simulink model "DSBSC_Modulation"  (R2021a)
settings: Solver=VariableStepAuto  StartTime=0.0  StopTime=10.0  RelTol=1e-3
libraries: dspfdesign x2
settings Model: Creator=ZephyrY  LastModifiedBy=ZephyrY

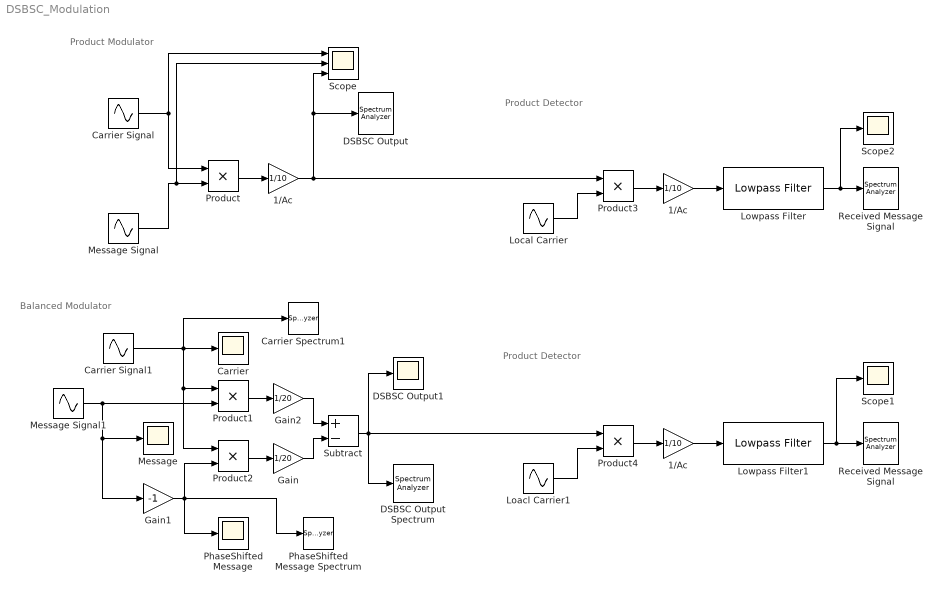
== system DSBSC_Modulation ==
  note: Product Detector
  note: Product Detector
  note: Product Modulator
  note: Balanced Modulator
  1/Ac : Gain  Gain=1/10
  "1/Ac " : Gain  Gain=1/10
  "1/Ac  " : Gain  Gain=1/10
  Carrier : Scope
  Carrier Signal : Sin  Amplitude=10  Frequency=2*pi*100  Phase=pi/2  SampleTime=1e-3
  Carrier Signal1 : Sin  Amplitude=10  Frequency=2*pi*100  Phase=pi/2  SampleTime=1e-3
  Carrier Spectrum1 : SpectrumAnalyzer
  DSBSC Output : SpectrumAnalyzer
  DSBSC Output Spectrum : SpectrumAnalyzer
  DSBSC Output1 : Scope
  Gain : Gain  Gain=1/20
  Gain1 : Gain  Gain=-1
  Gain2 : Gain  Gain=1/20
  Loacl Carrier1 : Sin  Amplitude=10  Frequency=2*pi*100  Phase=pi/2  SampleTime=1e-3
  Local Carrier : Sin  Amplitude=10  Frequency=2*pi*100  Phase=pi/2  SampleTime=1e-3
  Lowpass Filter : dspfdesign/Lowpass Filter  FilterType=FIR  DesignForMinimumOrder=off  FilterOrder=50  PassbandFrequency=15  StopbandFrequency=12e3  PassbandRipple=0.1  StopbandAttenuation=80  InheritSampleRate=on  SampleRate=44100  SimulateUsing=Interpreted execution  roundingMode=Floor  coeffsDataTypeStr=fixdt(1,16)
  Lowpass Filter1 : dspfdesign/Lowpass Filter  FilterType=FIR  DesignForMinimumOrder=off  FilterOrder=50  PassbandFrequency=15  StopbandFrequency=12e3  PassbandRipple=0.1  StopbandAttenuation=80  InheritSampleRate=on  SampleRate=44100  SimulateUsing=Interpreted execution  roundingMode=Floor  coeffsDataTypeStr=fixdt(1,16)
  Message : Scope
  Message Signal : Sin  Amplitude=5  Frequency=2*pi*10  Phase=pi/2  SampleTime=1e-3
  Message Signal1 : Sin  Amplitude=5  Frequency=2*pi*10  Phase=pi/2  SampleTime=1e-3
  PhaseShifted Message : Scope
  PhaseShifted Message Spectrum : SpectrumAnalyzer
  Product{,1..4} (5 alike) : Product
  Received Message Signal : SpectrumAnalyzer
  "Received Message Signal " : SpectrumAnalyzer
  Scope : Scope  NumInputPorts=3
  Scope1 : Scope
  Scope2 : Scope
  Subtract : Sum  Inputs=+-
  wires:
  Carrier Signal/1 -> Scope/1, Product/1
  Message Signal/1 -> Scope/2, Product/2
  Product/1 -> 1/Ac/1
  1/Ac/1 -> DSBSC Output/1, Scope/3, Product3/1
  Gain/1 -> Subtract/2
  Carrier Signal1/1 -> Carrier Spectrum1/1, Product1/1, Product2/1, Carrier/1
  Gain2/1 -> Subtract/1
  Subtract/1 -> DSBSC Output Spectrum/1, Product4/1, DSBSC Output1/1
  Gain1/1 -> PhaseShifted Message Spectrum/1, PhaseShifted Message/1, Product2/2
  Message Signal1/1 -> Product1/2, Gain1/1, Message/1
  Product1/1 -> Gain2/1
  Product2/1 -> Gain/1
  Local Carrier/1 -> Product3/2
  Loacl Carrier1/1 -> Product4/2
  Product3/1 -> "1/Ac  "/1
  Product4/1 -> "1/Ac "/1
  "1/Ac  "/1 -> Lowpass Filter/1
  "1/Ac "/1 -> Lowpass Filter1/1
  Lowpass Filter/1 -> Scope2/1, Received Message Signal/1
  Lowpass Filter1/1 -> Scope1/1, "Received Message Signal "/1
